simulink model "q_aero_2dof_control"  (R2024b)
settings: Solver=ode1  StartTime=0.0  StopTime=5  FixedStep=0.002  RelTol=1e-3  EnableMultiTasking=on
PreLoadFcn:
  | quanser_aero_parameters;
  | quanser_aero_state_space;
  | quanser_aero_lqr;
values from neighbouring files (symbols this model uses):
  A = [ 0           1            0            0 ... (first row only)    [quanser_aero_state_space.m]
  B = [ 0              0 ... (first row only)    [quanser_aero_state_space.m]
  C = [ 1  0  0  0 ... (first row only)    [quanser_aero_state_space.m]
  D = zeros(2,2)    [quanser_aero_state_space.m]
libraries: simulink x4, simulink_extras x2, quarc_library x2, quanser_aero x1
settings Model: SimulationMode=external  ExtModeTrigDuration=15000  Creator=MLevis  LastModifiedBy=niel
settings SolverCC: AlgebraicLoopSolver=TrustRegion  PositivePriorityOrder=on  AutoInsertRateTranBlk=on
settings DataIOCC: LimitDataPoints=on  SaveFormat=Array  ReturnWorkspaceOutputs=off
settings OptimizationCC: LifeSpan=inf
settings DebuggingCC: SolverPrmCheckMsg=warning  UnconnectedInputMsg=warning  UnconnectedOutputMsg=warning  UnconnectedLineMsg=warning  SFUnexpectedBacktrackingDiag=warning  SFNoUnconditionalDefaultTransitionDiag=warning  SFExecutionAtInitializationDiag=none  ArithmeticOperatorsInVariantConditions=warning
settings HardwareCC: ProdBitPerPointer=32  ProdBitPerSizeT=32  ProdBitPerPtrDiffT=32  ProdLargestAtomicFloat=None  ProdIntDivRoundTo=Undefined  ProdEndianess=Unspecified  ProdWordSize=32  ProdHWDeviceType=32-bit Generic
settings ModelReferenceCC: EnableRefExpFcnMdlSchedulingChecks=on  PropagateSignalLabelsOutOfModel=off
settings SFSimCC: SimUseLocalCustomCode=off  CustomCodeUndefinedFunction=UseInterfaceOnly  SimTargetLang=C++
settings RTWCC: Description=QUARC Win64 Target  SystemTargetFile=quarc_win64.tlc  MakeCommand="make_rtw OPTS=\" -D_USE_MATH_DEFINES  -D_USE_CXX11 \""  TemplateMakefile=quarc_default_tmf  RTWUseLocalCustomCode=off  CustomInclude=C:\Users\philippe\Desktop\quanser-aero-tp-instructor\simulink\..\quanser-aero-tp\simulink\quanser-aero-mpc\src C:\Users\philippe\Desktop\quanser-aero-tp-instructor\simulink\..\quanser-aero-tp\simulink\quanser-aero-mpc\3d_party C:\Users\philippe\Desktop\quanser-aero-tp-instructor\simulink\..\quanser-aero-tp\simulink\quanser-aero-mpc\3d_party\eigen3 C:\Users\philippe\Desktop\quanser-aero-tp-instructor\simulink\..\quanser-aero-tp\simulink\quanser-aero-mpc\3d_party\polympc C:\Users\philippe\Desktop\quanser-aero-tp-instructor\simulink\..\quanser-aero-tp\simulink\quanser-aero-mpc\3d_party\polympc\src  TargetLang=C++  GPUComputeCapability=3.5
settings CodeAppCC: StateflowObjectComments=on
settings STFCustomTargetCC: TargetPreCompLibLocation=C:\PROGRA~3\QUARC\lib\2019b\win64\release  TargetLangStandard=C++03 (ISO)  ConcurrentExecutionCompliant=on  GRTInterface=on  SystemTargetFile=quarc_win64.tlc
settings GRTTargetCC: TargetPreCompLibLocation=C:\PROGRA~3\QUARC\lib\2019b\win64\release  TargetLangStandard=C++03 (ISO)  ParMdlRefBuildCompliant=off  CompOptLevelCompliant=off  CombineOutputUpdateFcns=off  MatFileLogging=off  CPPClassGenCompliant=off  GRTInterface=on  UseToolchainInfoCompliant=off  ExtMode=on  ExtModeMexFile=quarc_comm
settings ConfigComp: CovMetricSettings=dw  CovSaveCumulativeToWorkspaceVar=on  CovSaveSingleToWorkspaceVar=on  CovExternalEMLEnable=off  CovSFcnEnable=off

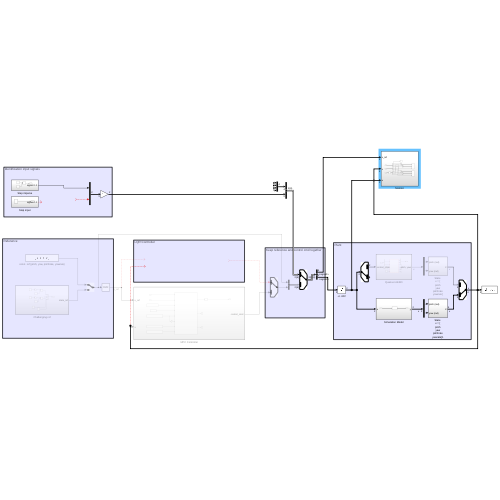
[thumbnail: Simulink's stored preview of the top-level diagram]
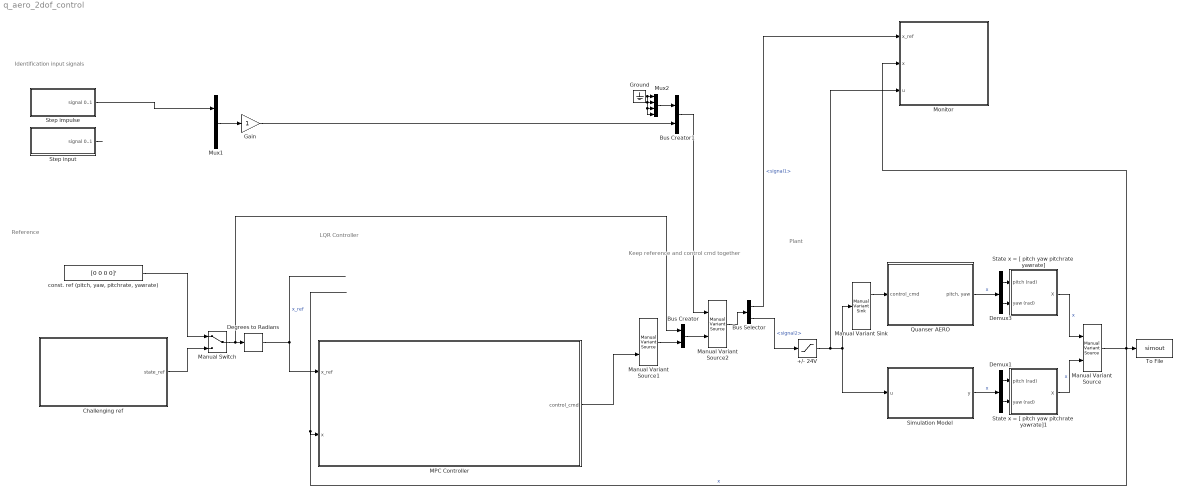
== system q_aero_2dof_control ==
  note: Keep reference and control cmd together
  note: LQR Controller
  note: Reference
  note: Identification input signals
  note: Plant
  +/- 24V : Saturate  UpperLimit=24  LowerLimit=-24
  Bus Creator : BusCreator  Inputs=2
  Bus Creator1 : BusCreator  Inputs=2
  Bus Selector : BusSelector  OutputSignals=signal1,signal2
  Challenging ref : Subsystem
  Degrees to Radians : simulink_extras/Transformations/Degrees to Radians
  Demux1 : Demux  Outputs=2
  Demux3 : Demux  Outputs=2
  Gain : Gain
  Ground : Ground
  MPC Controller : Subsystem
  Manual Variant Sink : simulink/Signal Routing/Manual Variant Sink  NumChoices=2  LabelModeActiveChoice=V_2
  Manual Variant Source : simulink/Signal Routing/Manual Variant Source  NumChoices=2  LabelModeActiveChoice=V_2
  Manual Variant Source1 : simulink/Signal Routing/Manual Variant Source  NumChoices=2  LabelModeActiveChoice=V_1
  Manual Variant Source2 : simulink/Signal Routing/Manual Variant Source  NumChoices=2  LabelModeActiveChoice=V_1
  Manual Switch : ManualSwitch
  Monitor : Subsystem
  Mux1 : Mux  Inputs=2
  Mux2 : Mux
  Quanser AERO : Subsystem
  Simulation Model : Subsystem
  State x = [ pitch yaw pitchrate yawrate] : Subsystem
  State x = [ pitch yaw pitchrate yawrate]1 : Subsystem
  Step impulse : Subsystem
  Step input : Subsystem
  To File : ToFile  Filename=simout
  "const. ref (pitch, yaw, pitchrate, yawrate)" : Constant  Value=[0 0 0 0]'
  wires:
  Manual Variant Source/1 -> Monitor/2(x), MPC Controller/2(x), To File/1  "x"
  Mux2/1 -> Bus Creator1/1
  ? -> Manual Variant Source1/1
  Bus Selector/1 -> Monitor/1(x_ref)  "<signal1>"
  Bus Creator/1 -> Manual Variant Source2/2
  "const. ref (pitch, yaw, pitchrate, yawrate)"/1 -> Manual Switch/1
  Challenging ref/1(state_ref) -> Manual Switch/2
  MPC Controller/1("control_cmd ") -> Manual Variant Source1/2
  Manual Variant Source2/1 -> Bus Selector/1
  Bus Creator1/1 -> Manual Variant Source2/1
  Manual Variant Source1/1 -> Bus Creator/2
  Degrees to Radians/1 -> MPC Controller/1(x_ref)  "x_ref"
  Ground/1 -> Mux2/1, Mux2/4, Mux2/3, Mux2/2
  Manual Switch/1 -> Bus Creator/1, Degrees to Radians/1
  Gain/1 -> Bus Creator1/2
  Mux1/1 -> Gain/1
  ? -> Mux1/2
  Step input/1(signal 0..1) -> ?
  Demux3/1 -> State x = [ pitch yaw pitchrate yawrate]/1(pitch (rad))
  Quanser AERO/1("pitch, yaw") -> Demux3/1  "x"
  +/- 24V/1 -> Monitor/3(u), Simulation Model/1(u), Manual Variant Sink/1
  Manual Variant Sink/1 -> Quanser AERO/1(control_cmd)
  Simulation Model/1(y) -> Demux1/1  "x"
  Demux3/2 -> State x = [ pitch yaw pitchrate yawrate]/2(yaw (rad))
  Demux1/1 -> State x = [ pitch yaw pitchrate yawrate]1/1(pitch (rad))
  State x = [ pitch yaw pitchrate yawrate]1/1(X) -> Manual Variant Source/2  "x"
  Demux1/2 -> State x = [ pitch yaw pitchrate yawrate]1/2(yaw (rad))
  Bus Selector/2 -> +/- 24V/1  "<signal2>"
  State x = [ pitch yaw pitchrate yawrate]/1(X) -> Manual Variant Source/1  "x"
  Step impulse/1(signal 0..1) -> Mux1/1

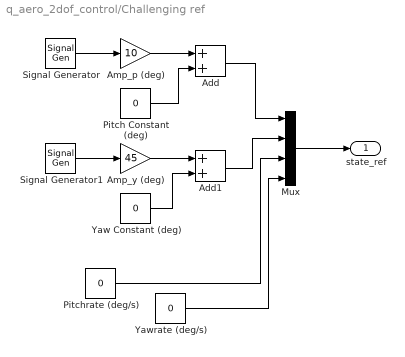
== system q_aero_2dof_control/Challenging ref ==
  Add : Sum
  Add1 : Sum
  Amp_p (deg) : Gain  Gain=10
  Amp_y (deg) : Gain  Gain=45
  Mux : Mux
  Pitch Constant (deg) : Constant  Value=0
  Pitchrate (deg/s) : Constant  Value=0
  Signal Generator : SignalGenerator  WaveForm=square  Frequency=0.1
  Signal Generator1 : SignalGenerator  WaveForm=square  Frequency=0.04
  Yaw Constant (deg) : Constant  Value=0
  Yawrate (deg/s) : Constant  Value=0
  state_ref : Outport
  wires:
  Add/1 -> Mux/1
  Amp_p (deg)/1 -> Add/1
  Signal Generator1/1 -> Amp_y (deg)/1
  Mux/1 -> state_ref/1
  Yaw Constant (deg)/1 -> Add1/2
  Add1/1 -> Mux/2
  Signal Generator/1 -> Amp_p (deg)/1
  Pitchrate (deg/s)/1 -> Mux/3
  Yawrate (deg/s)/1 -> Mux/4
  Amp_y (deg)/1 -> Add1/1
  Pitch Constant (deg)/1 -> Add/2

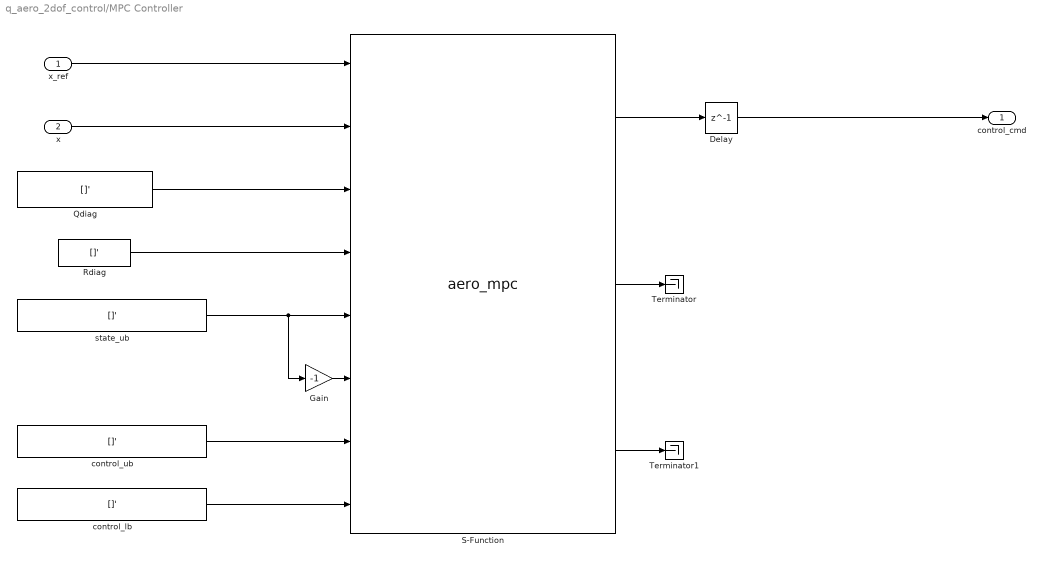
== system q_aero_2dof_control/MPC Controller ==
  x_ref : Inport
  x : Inport  Port=2
  Delay : Delay  DelayLength=1  InitialCondition=[0 0 0 0]'
  Gain : Gain  Gain=-1
  Qdiag : Constant  Value=[]'
  Rdiag : Constant  Value=[]'
  S-Function : S-Function  FunctionName=aero_mpc  Parameters=Ampc, Bmpc  SFunctionModules=aero_mpc_wrapper  SFunctionDeploymentMode=off  EnableBusSupport=off
      mask Display:
      | text(0.5, 0.5, 'PolyMPC Tracking Controller\n\ndim(x) = dim(u) = 4', 'horizontalAlignment', 'center')
      | 
      | port_label('input', 1, 'state_ref')
      | port_label('input', 2, 'state')
      | port_label('input', 3, 'Qdiag')
      | port_label('input', 4, 'Rdiag')
      | port_label('input', 5, 'state_ub')
      | port_label('input', 6, 'state_lb')
      | port_label('input', 7, 'control_ub')
      | port_label('input', 8, 'control_lb')
      | 
      | port_label('output', 1, 'control_cmd')
      | port_label('output', 2, 'solve_status')
      | port_label('output', 3, 'comp_time_us')
  Terminator : Terminator
  Terminator1 : Terminator
  control_lb : Constant  Value=[]'
  control_ub : Constant  Value=[]'
  state_ub : Constant  Value=[]'
  "control_cmd " : Outport
  wires:
  Rdiag/1 -> S-Function/4
  Qdiag/1 -> S-Function/3
  Delay/1 -> "control_cmd "/1
  state_ub/1 -> Gain/1, S-Function/5
  Gain/1 -> S-Function/6
  control_lb/1 -> S-Function/8
  S-Function/3 -> Terminator1/1
  S-Function/2 -> Terminator/1
  control_ub/1 -> S-Function/7
  S-Function/1 -> Delay/1
  x_ref/1 -> S-Function/1
  x/1 -> S-Function/2

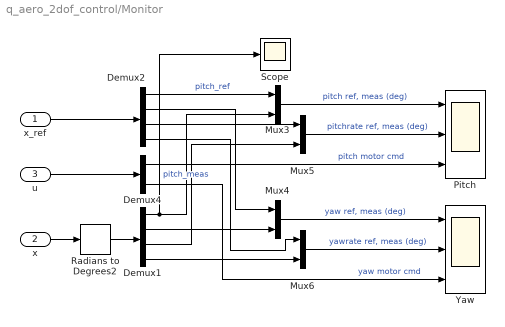
== system q_aero_2dof_control/Monitor ==
  x_ref : Inport
  x : Inport  Port=2
  u : Inport  Port=3
  Demux1 : Demux
  Demux2 : Demux
  Demux4 : Demux  Outputs=2
  Mux{3..6} (4 alike) : Mux  Inputs=2
  Pitch : Scope  NumInputPorts=3
  Radians to Degrees2 : simulink_extras/Transformations/Radians to Degrees
  Scope : Scope
  Yaw : Scope  NumInputPorts=3
  wires:
  Demux1/3 -> Mux5/2
  Demux1/2 -> Mux4/2
  Demux1/4 -> Mux6/2
  Demux2/4 -> Mux6/1
  Demux1/1 -> Scope/1, Mux3/2  "pitch_meas"
  Demux2/3 -> Mux5/1
  Demux2/1 -> Mux3/1  "pitch_ref"
  Mux3/1 -> Pitch/1  "pitch ref, meas (deg)"
  Mux4/1 -> Yaw/1  "yaw ref, meas (deg)"
  Mux5/1 -> Pitch/2  "pitchrate ref, meas (deg)"
  Demux4/1 -> Pitch/3  "pitch motor cmd"
  Demux4/2 -> Yaw/3  "yaw motor cmd"
  Demux2/2 -> Mux4/1
  Radians to Degrees2/1 -> Demux1/1
  u/1 -> Demux4/1
  Mux6/1 -> Yaw/2  "yawrate ref, meas (deg)"
  x/1 -> Radians to Degrees2/1
  x_ref/1 -> Demux2/1

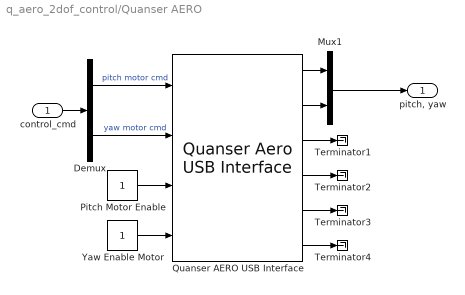
== system q_aero_2dof_control/Quanser AERO ==
  control_cmd : Inport
  Demux : Demux  Outputs=2
  Mux1 : Mux  Inputs=2
  Pitch Motor Enable : Constant
  Quanser AERO USB Interface : quanser_aero/Quanser Aero USB Interface  SystemSampleTime=-1  Latency=0  AutoFrameSizeCalculation=off
      link override HIL Write: analog_channels=[0;1]
  Terminator{1..4} (4 alike) : Terminator
  Yaw Enable Motor : Constant
  "pitch, yaw" : Outport
  wires:
  Pitch Motor Enable/1 -> Quanser AERO USB Interface/3
  Quanser AERO USB Interface/4 -> Terminator2/1
  Yaw Enable Motor/1 -> Quanser AERO USB Interface/4
  Quanser AERO USB Interface/5 -> Terminator3/1
  Demux/2 -> Quanser AERO USB Interface/2  "yaw motor cmd"
  Quanser AERO USB Interface/2 -> Mux1/2
  Demux/1 -> Quanser AERO USB Interface/1  "pitch motor cmd"
  Quanser AERO USB Interface/6 -> Terminator4/1
  Quanser AERO USB Interface/1 -> Mux1/1
  Quanser AERO USB Interface/3 -> Terminator1/1
  Mux1/1 -> "pitch, yaw"/1
  control_cmd/1 -> Demux/1

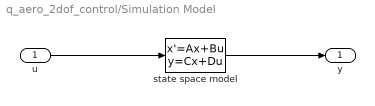
== system q_aero_2dof_control/Simulation Model ==
  u : Inport
  state space model : StateSpace  A=A  B=B  C=C  D=D  InitialCondition=0
  y : Outport
  wires:
  u/1 -> state space model/1
  state space model/1 -> y/1

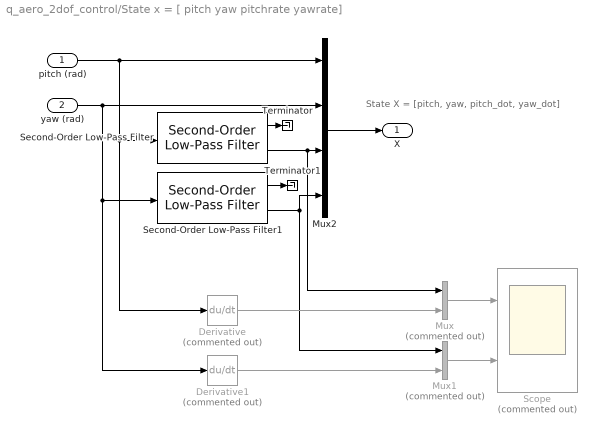
== system q_aero_2dof_control/State x = [ pitch yaw pitchrate yawrate] ==
  note: State X = [pitch, yaw, pitch_dot, yaw_dot]
  pitch (rad) : Inport
  yaw (rad) : Inport  Port=2
  Derivative : Derivative  Commented=on
  Derivative1 : Derivative  Commented=on
  Mux : Mux  Commented=on  Inputs=2
  Mux1 : Mux  Commented=on  Inputs=2
  Mux2 : Mux
  Scope : Scope  Commented=on  NumInputPorts=2
  Second-Order Low-Pass Filter : quarc_library/Continuous/Second-Order Low-Pass Filter  params_source=Internal (dialog parameters)  input_width=50  input_zeta=0.8  input_init=0
  Second-Order Low-Pass Filter1 : quarc_library/Continuous/Second-Order Low-Pass Filter  params_source=Internal (dialog parameters)  input_width=50  input_zeta=0.8  input_init=0
  Terminator : Terminator
  Terminator1 : Terminator
  X : Outport
  wires:
  Mux2/1 -> X/1
  yaw (rad)/1 -> Derivative1/1, Second-Order Low-Pass Filter1/1, Mux2/2
  pitch (rad)/1 -> Second-Order Low-Pass Filter/1, Derivative/1, Mux2/1
  Second-Order Low-Pass Filter/2 -> Mux/1, Mux2/3
  Second-Order Low-Pass Filter1/2 -> Mux2/4, Mux1/1
  Second-Order Low-Pass Filter/1 -> Terminator/1
  Second-Order Low-Pass Filter1/1 -> Terminator1/1
  Derivative/1 -> Mux/2
  Mux/1 -> Scope/1
  Derivative1/1 -> Mux1/2
  Mux1/1 -> Scope/2

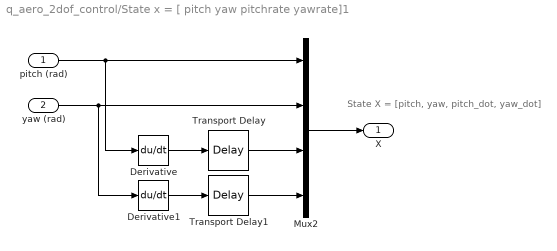
== system q_aero_2dof_control/State x = [ pitch yaw pitchrate yawrate]1 ==
  note: State X = [pitch, yaw, pitch_dot, yaw_dot]
  pitch (rad) : Inport
  yaw (rad) : Inport  Port=2
  Derivative : Derivative
  Derivative1 : Derivative
  Mux2 : Mux
  Transport Delay : TransportDelay  DelayTime=0.03
  Transport Delay1 : TransportDelay  DelayTime=0.03
  X : Outport
  wires:
  Mux2/1 -> X/1
  yaw (rad)/1 -> Derivative1/1, Mux2/2
  pitch (rad)/1 -> Derivative/1, Mux2/1
  Derivative/1 -> Transport Delay/1
  Derivative1/1 -> Transport Delay1/1
  Transport Delay/1 -> Mux2/3
  Transport Delay1/1 -> Mux2/4

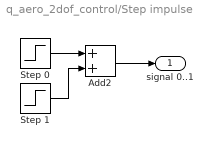
== system q_aero_2dof_control/Step impulse ==
  Add2 : Sum
  Step 0 : Step  SampleTime=0
  Step 1 : Step  Time=1.75  After=-1  SampleTime=0
  signal 0..1 : Outport
  wires:
  Add2/1 -> signal 0..1/1
  Step 1/1 -> Add2/2
  Step 0/1 -> Add2/1

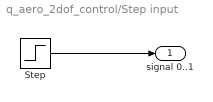
== system q_aero_2dof_control/Step input ==
  Step : Step  SampleTime=0
  signal 0..1 : Outport
  wires:
  Step/1 -> signal 0..1/1
